simulink model "VSI"  (R2019a)
settings: Solver=VariableStepAuto  StartTime=0.0  StopTime=10.0  RelTol=1e-3  EnableMultiTasking=on
values from neighbouring files (symbols this model uses):
  e = 100    [Parameters.m]
  f_e = 50    [Parameters.m]
  f_ref = 50    [Parameters.m]
  I_ref_peak = 10    [Parameters.m]
  L = 10e-3    (= 0.01)    [Parameters.m]
  R = 10    [Parameters.m]
libraries: powerlib x12, eeTransforms x2, powerlib_meascontrol x1
settings Model: Creator=The MathWorks, Inc.  LastModifiedBy=pc
settings DataIOCC: LimitDataPoints=on  ReturnWorkspaceOutputs=off
settings OptimizationCC: LifeSpan=inf
settings DebuggingCC: AllowSymbolicDim=off  SFUnexpectedBacktrackingDiag=warning  SFNoUnconditionalDefaultTransitionDiag=warning  SFExecutionAtInitializationDiag=none  ArithmeticOperatorsInVariantConditions=warning
settings ModelReferenceCC: PropagateSignalLabelsOutOfModel=off
settings SFSimCC: SimUseLocalCustomCode=off
settings RTWCC: RTWUseLocalCustomCode=off
settings CodeAppCC: StateflowObjectComments=on
settings GRTTargetCC: TargetLangStandard=C89/C90 (ANSI)
settings ConfigComp: CovMetricSettings=dw  CovHtmlReporting=on  CovSaveCumulativeToWorkspaceVar=on  CovSaveSingleToWorkspaceVar=on  CovExternalEMLEnable=off

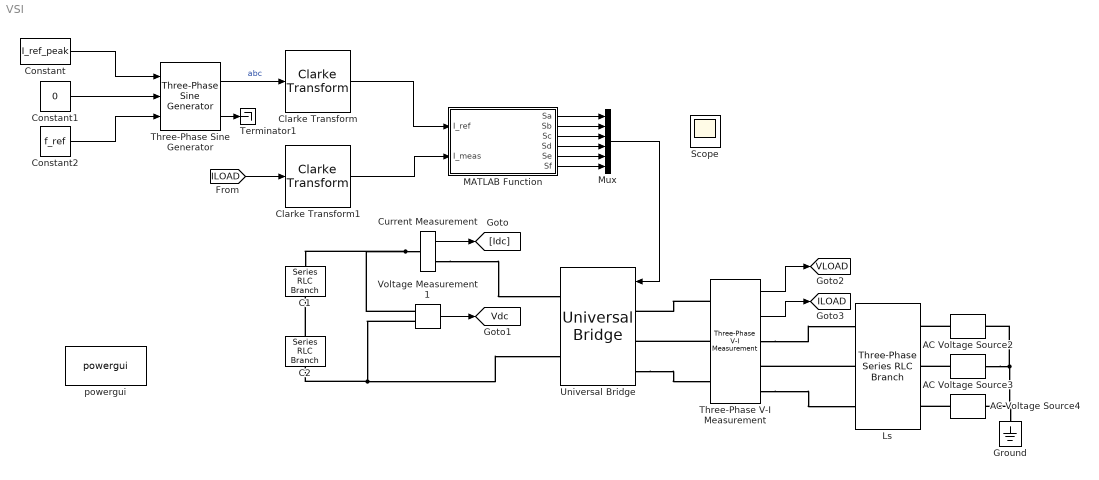
== system VSI ==
  AC Voltage Source2 : powerlib/Electrical Sources/AC Voltage Source  Amplitude=e  Phase=0  Frequency=f_e  SampleTime=0  Measurements=None  BusType=swing  Pref=10e3  Qref=0  Qmin=-inf  Qmax=+inf
      settings: SourceProductName=Simscape Electrical
  AC Voltage Source3 : powerlib/Electrical Sources/AC Voltage Source  Amplitude=e  Phase=-120  Frequency=f_e  SampleTime=0  Measurements=None  BusType=swing  Pref=10e3  Qref=0  Qmin=-inf  Qmax=+inf
      settings: SourceProductName=Simscape Electrical
  AC Voltage Source4 : powerlib/Electrical Sources/AC Voltage Source  Amplitude=e  Phase=120  Frequency=f_e  SampleTime=0  Measurements=None  BusType=swing  Pref=10e3  Qref=0  Qmin=-inf  Qmax=+inf
      settings: SourceProductName=Simscape Electrical
  C1 : powerlib/Elements/Series RLC Branch  LConnTagsString=__new0  RConnTagsString=__new0  BranchType=C  Resistance=1  Inductance=1e-3  SetiL0=off  InitialCurrent=0  Capacitance=5  Setx0=off  InitialVoltage=0  Measurements=None
      settings: SourceProductName=Simscape Electrical
  C2 : powerlib/Elements/Series RLC Branch  LConnTagsString=__new0  RConnTagsString=__new0  BranchType=C  Resistance=1  Inductance=1e-3  SetiL0=off  InitialCurrent=0  Capacitance=5  Setx0=off  InitialVoltage=0  Measurements=None
      settings: SourceProductName=Simscape Electrical
  Clarke Transform : eeTransforms/Clarke Transform  PowerInvariant=off
      settings: SourceProductName=Simscape Electrical  SourceProductBaseCode=PS
  Clarke Transform1 : eeTransforms/Clarke Transform  PowerInvariant=off
      settings: SourceProductName=Simscape Electrical  SourceProductBaseCode=PS
  Constant : Constant  Value=I_ref_peak
  Constant1 : Constant  Value=0
  Constant2 : Constant  Value=f_ref
  Current Measurement : powerlib/Measurements/Current Measurement  PhasorSimulation=off  OutputType=Complex  PSBequivalent=0
      settings: SourceProductName=Simscape Electrical
  Ground : powerlib/Elements/Ground  LConnTagsString=a
      settings: SourceProductName=Simscape Electrical
  Ls : powerlib/Elements/Three-Phase Series RLC Branch  LConnTagsString=A|B|C  RConnTagsString=A|B|C  BranchType=RL  Resistance=R  Inductance=L  Capacitance=1e-6  Measurements=None
      settings: SourceProductName=Simscape Electrical
  MATLAB Function : MATLAB Function  TreatAsAtomicUnit=on
  Mux : Mux  Inputs=6
  Scope : Scope
  Terminator1 : Terminator
  Three-Phase Sine Generator : powerlib_meascontrol/Pulse & Signal Generators/Three-Phase Sine Generator  Ts=0
      settings: SourceProductName=Simscape Electrical  SourceProductBaseCode=PS
  Three-Phase V-I Measurement : powerlib/Measurements/Three-Phase V-I Measurement  VoltageMeasurement=phase-to-ground  SetLabelV=off  LabelV=Vabc  Vpu=off  VpuLL=off  CurrentMeasurement=yes  SetLabelI=off  LabelI=Iabc  Ipu=off  Pbase=100e6  Vbase=500e3  OutputType=Complex  PhasorSimulation=off  PSBequivalent=0
      settings: SourceProductName=Simscape Electrical
  Universal Bridge : powerlib/Power Electronics/Universal Bridge  Arms=3  SnubberResistance=1e5  SnubberCapacitance=inf  Device=IGBT / Diodes  Ron=1e-3  Lon=0  ForwardVoltages="[  0  0  ]"  ForwardVoltage=0  GTOparameters=[ 10e-6 , 20e-6 ]  IGBTparameters=[ 1e-6 , 2e-6 ]  Measurements=None  Measurements_2=None  converterType=Rectifier
      settings: SourceProductName=Simscape Electrical
  Voltage Measurement1 : powerlib/Measurements/Voltage Measurement  PhasorSimulation=off  OutputType=Complex  PSBequivalent=0
      settings: SourceProductName=Simscape Electrical
  powergui : powerlib/powergui  Priority=1  SimulationMode=Continuous  SampleTime=50e-6  frequency=60  Iterations=50  frequencyindice=50  Pbase=100e6  ErrMax=1e-4  UnitsV=kV  UnitsW=MW  buscounter=0  FunctionMessages=off  echomessages=off  EnableUseOfTLC=off  CurrentSourceSwitches=off  DisableSnubberDevices=off  DisableRonSwitches=off  DisableVfSwitches=off  DisplayEquations=off  AutomaticDiscreteSolvers=off  SolverType=Tustin/Backward Euler (TBE)  Interpol=off  ExternalGateDelay=off  methode=off  Ts=100  x0status=blocks  SPID=on  SwTol=0  HookPort=off  NonlinearTolerance=0  nMaxIteration=15  ContinueOnMaxIteration=off  RestoreLinks=warning  ResistiveCurrentMeasurement=off  Frange=[0:2:500]  Ylog=off  Xlog=on  ShowGrid=off  save=off  variable=ZData  structure=0  ZoomFFT=off  StartTime=0.0  cycles=1  DisplayStyle=1  fundamental=60  FreqAxis=off  MaxFrequency=1000  frequencyindicesteady=1  RmsSteady=1  display=off
      settings: SourceProductName=Simscape Electrical
  tag scope: ILOAD=global, VLOAD=global, Vdc=global
  wires:
  Voltage Measurement1/1 -> [Vdc]
  Current Measurement/1 -> [Idc]
  Three-Phase V-I Measurement/2 -> [ILOAD]
  Three-Phase V-I Measurement/1 -> [VLOAD]
  Three-Phase Sine Generator/1 -> Clarke Transform/1  "abc"
  Three-Phase Sine Generator/2 -> Terminator1/1
  [ILOAD] -> Clarke Transform1/1
  Constant1/1 -> Three-Phase Sine Generator/2
  Constant/1 -> Three-Phase Sine Generator/1
  Clarke Transform/1 -> MATLAB Function/1(I_ref)
  Constant2/1 -> Three-Phase Sine Generator/3
  Clarke Transform1/1 -> MATLAB Function/2(I_meas)
  MATLAB Function/1(Sa) -> Mux/1
  MATLAB Function/2(Sb) -> Mux/2
  MATLAB Function/3(Sc) -> Mux/3
  MATLAB Function/4(Sd) -> Mux/4
  MATLAB Function/5(Se) -> Mux/5
  MATLAB Function/6(Sf) -> Mux/6
  Mux/1 -> Universal Bridge/1
  connections:
  Current Measurement/LConn1 -- Voltage Measurement1/LConn1 -- C1/LConn1
  Voltage Measurement1/LConn2 -- C2/RConn1 -- Universal Bridge/RConn2
  Current Measurement/RConn1 -- Universal Bridge/RConn1
  C2/LConn1 -- C1/RConn1
  AC Voltage Source3/LConn1 -- Ground/LConn1 -- AC Voltage Source4/LConn1 -- AC Voltage Source2/LConn1
  AC Voltage Source4/RConn1 -- Ls/LConn3
  AC Voltage Source3/RConn1 -- Ls/LConn2
  AC Voltage Source2/RConn1 -- Ls/LConn1
  Three-Phase V-I Measurement/LConn2 -- Universal Bridge/LConn2
  Three-Phase V-I Measurement/LConn1 -- Universal Bridge/LConn1
  Universal Bridge/LConn3 -- Three-Phase V-I Measurement/LConn3
  Three-Phase V-I Measurement/RConn1 -- Ls/RConn1
  Ls/RConn2 -- Three-Phase V-I Measurement/RConn2
  Three-Phase V-I Measurement/RConn3 -- Ls/RConn3

== matlab function VSI/MATLAB Function ==
  data: I_ref input; Sa output; I_meas input; Sb output; Sc output; Sd output; Se output; Sf output
function [Sa,Sb,Sc,Sd,Se,Sf] = control(I_ref,I_meas)
% Variables defined in the parameters file
global Ts R L v states
% Optimum vector and measured current at instant k-1
persistent x_old i_old
% Initialize values
if isempty(x_old), x_old = 1; end
if isempty(i_old), i_old = 0+1j*0; end
g_opt = 1e10;
% Read current reference inputs at sampling instant k
ik_ref = I_ref(1) + 1j*I_ref(2);
% Read current measurements at sampling instant k
ik = I_meas(1) + 1j*I_meas(2);
% Back-EMF estimate
e = v(x_old) - L/Ts*ik - (R - L/Ts)*i_old;
% Store the measured current for the next iteration
i_old = ik;
for i = 1:8
    % i-th voltage vector for current prediction
    v_o1 = v(i);
    % Current prediction at instant k+1
    ik1 = (1 - R*Ts/L)*ik + Ts/L*(v_o1 - e);
    % Cost function
    g = abs(real(ik_ref - ik1)) + abs(imag(ik_ref - ik1));
    % Selection of the optimal value
    if (g<g_opt)
        g_opt = g;
        x_opt = i;
    end
end
% Store the present value of x_opt
x_old = x_opt;
% Output switching states
Sa = states(x_opt,1);
Sb = ~Sa;
Sc = states(x_opt,2);
Sd = ~Sc;
Se = states(x_opt,3);
Sf = ~Se;
